simulink model "FF_statefbk"  (R2020b)
settings: Solver=ode45  StartTime=0.0  StopTime=120  RelTol=1e-3  EnableMultiTasking=on
values from neighbouring files (symbols this model uses):
  A = [0 1 ... (first row only)    [TestDIST_EFFECT_DCmotor_zp.m]
  B = [0; Kt/Rm/Jt]    [TestDIST_EFFECT_DCmotor_zp.m]
  Jt = Jm+J1+J2    (= 2.089856e-05)    [TestDIST_EFFECT_DCmotor_zp.m]
  KK = dlqr(Fs,Gs,Q,R)    [TestDIST_EFFECT_DCmotor_zp.m]
  Kt = 0.042    [TestDIST_EFFECT_DCmotor_zp.m]
  Rm = 8.4    [TestDIST_EFFECT_DCmotor_zp.m]
settings Model: Creator=oboe  LastModifiedBy=oboe
settings DataIOCC: LimitDataPoints=on  SaveFormat=Array  ReturnWorkspaceOutputs=off
settings OptimizationCC: LifeSpan=inf
settings DebuggingCC: SolverPrmCheckMsg=warning  SFUnexpectedBacktrackingDiag=warning  SFNoUnconditionalDefaultTransitionDiag=warning  SFExecutionAtInitializationDiag=none  ArithmeticOperatorsInVariantConditions=warning
settings HardwareCC: ProdBitPerPointer=32  ProdBitPerSizeT=32  ProdBitPerPtrDiffT=32  ProdLargestAtomicFloat=None  ProdIntDivRoundTo=Undefined  ProdEndianess=Unspecified  ProdWordSize=32  ProdHWDeviceType=32-bit Generic
settings ModelReferenceCC: PropagateSignalLabelsOutOfModel=off
settings SFSimCC: SimUseLocalCustomCode=off  CustomCodeUndefinedFunction=UseInterfaceOnly
settings RTWCC: RTWUseLocalCustomCode=off
settings CodeAppCC: StateflowObjectComments=on
settings GRTTargetCC: TargetLangStandard=C89/C90 (ANSI)
settings ConfigComp: CovMetricSettings=dw  CovSaveCumulativeToWorkspaceVar=on  CovSaveSingleToWorkspaceVar=on  CovExternalEMLEnable=off  CovSFcnEnable=off

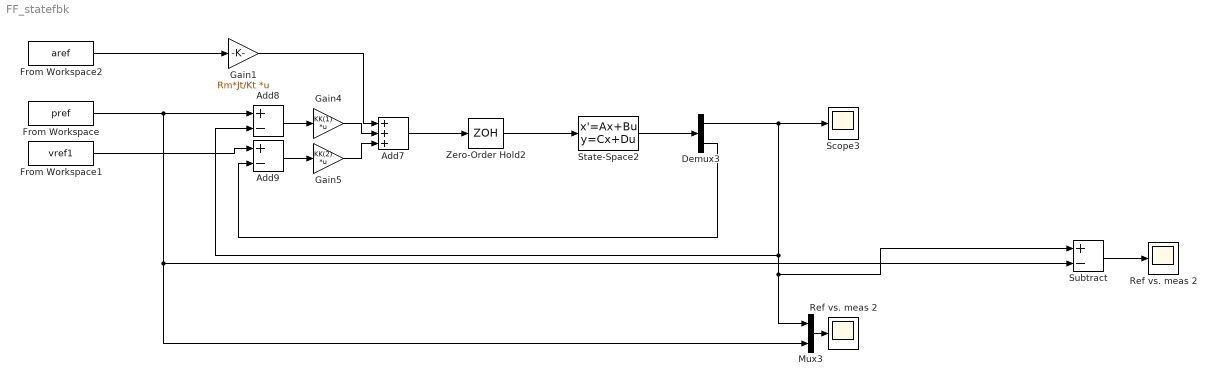
== system FF_statefbk ==
  Add7 : Sum  Inputs=+++
  Add8 : Sum  Inputs=+-
  Add9 : Sum  Inputs=+-
  Demux3 : Demux  Outputs=2
  From Workspace : FromWorkspace  VariableName=pref
  From Workspace1 : FromWorkspace  VariableName=vref1
  From Workspace2 : FromWorkspace  VariableName=aref
  Gain1 : Gain  Gain=Rm*Jt/Kt  Multiplication=Matrix(K*u)
  Gain4 : Gain  Gain=KK(1)  Multiplication=Matrix(K*u)
  Gain5 : Gain  Gain=KK(2)  Multiplication=Matrix(K*u)
  Mux3 : Mux  Inputs=2
  Ref vs. meas 2 : Scope
  "Ref vs. meas 2 " : Scope
  Scope3 : Scope
  State-Space2 : StateSpace  A=A(1:2,1:2)  B=B(1:2)  C=eye(2)  D=[0;0]  InitialCondition=0
  Subtract : Sum  Inputs=+-
  Zero-Order Hold2 : ZeroOrderHold  SampleTime=0.001
  wires:
  Mux3/1 -> "Ref vs. meas 2 "/1
  Zero-Order Hold2/1 -> State-Space2/1
  Demux3/1 -> Add8/2, Subtract/1, Mux3/1, Scope3/1
  Gain4/1 -> Add7/2
  Add7/1 -> Zero-Order Hold2/1
  Gain5/1 -> Add7/3
  State-Space2/1 -> Demux3/1
  Demux3/2 -> Add9/2
  Add9/1 -> Gain5/1
  Add8/1 -> Gain4/1
  From Workspace/1 -> Add8/1, Mux3/2, Subtract/2
  Subtract/1 -> Ref vs. meas 2/1
  From Workspace1/1 -> Add9/1
  From Workspace2/1 -> Gain1/1
  Gain1/1 -> Add7/1
